simulink model "OperatingMode_PLCCoder"  (R2024b)
settings: Solver=FixedStepAuto  StartTime=0.0  StopTime=2  FixedStep=0.1  MaxStep=TsModel  RelTol=1e-3
undefined symbols (not defined in the file): operatingMode
libraries: simulink x3
settings Model: DataDictionary=LocalDataD_SupervisoryLogic.sldd  Creator=vlenzi  LastModifiedBy=vlenzi
settings SolverCC: AlgebraicLoopSolver=TrustRegion
settings OptimizationCC: DefaultParameterBehavior=Inlined  ReuseModelBlockBuffer=off
settings DebuggingCC: InheritedTsInSrcMsg=none  UnconnectedInputMsg=warning  UnconnectedOutputMsg=warning  UnconnectedLineMsg=warning
settings ModelReferenceCC: EnableRefExpFcnMdlSchedulingChecks=on
settings RTWCC: GPUComputeCapability=3.5  DLArmComputeVersion=19.05
settings ConfigComp: PLC_OutputDir=..\Code\plcsrc  PLC_TargetIDE=twincat3  PLC_GenerateTestbench=on  PLC_GenerateTestbenchDiagCode=on  PLC_MultiTBSigbuilderTimeRange=off  PLC_GenerateReusableCode=on  PLC_InlineNamedConstant=on  PLC_FoldFBCallOutputVar=on  PLC_RemoveUnusedSSMethodCallArguments=on  PLC_FBUseSubsystemInstanceName=on  PLC_RemoveTopFBSSMethodType=on  PLC_UseCallOutputArgSyntax=off  PLC_OverrideDefaultNameLength=on  PLC_EnableUnsignedAndDoubleTypes=off  PLC_EnableUDTSplitting=off  PLC_MaxFieldsInUDT=500  PLC_GenerateEnumCastFunction=on  PLC_InlineEnumCastFunction=off  PLC_RTWMaxIdLength=64  PLC_GenerateWebView=on

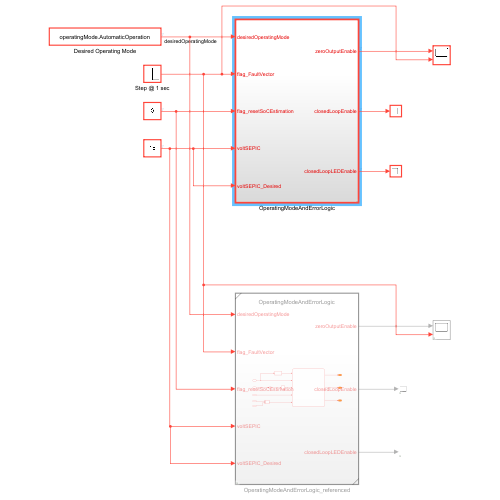
[thumbnail: Simulink's stored preview of the top-level diagram]
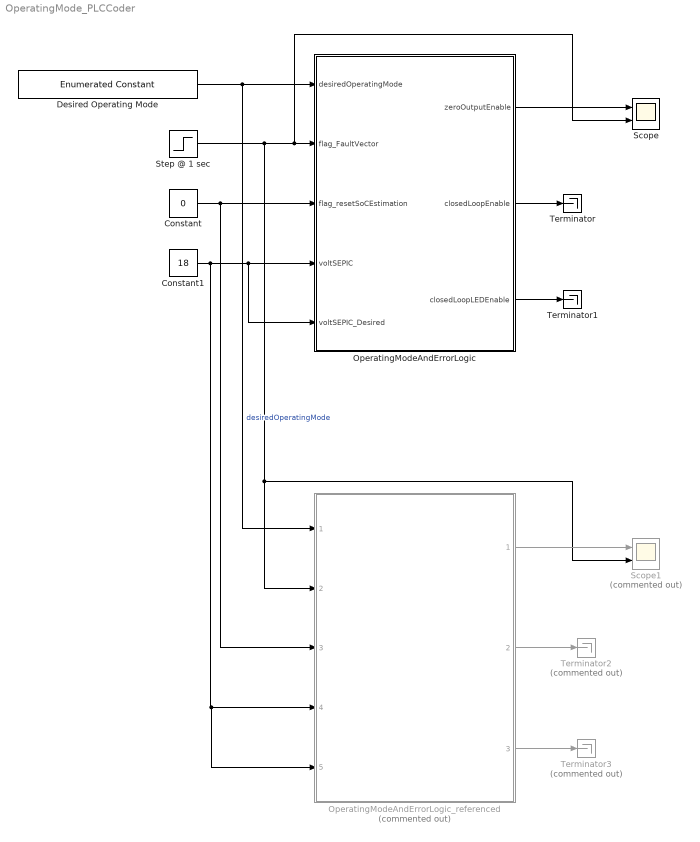
== system OperatingMode_PLCCoder ==
  Constant : Constant  Value=0  OutDataTypeStr=boolean  SampleTime=-1
  Constant1 : Constant  Value=18  SampleTime=-1
  Desired Operating Mode : simulink/Sources/Enumerated Constant  OutDataTypeStr=Enum: operatingMode  Value=operatingMode.AutomaticOperation  SampleTime=-1
  OperatingModeAndErrorLogic : Subsystem  TreatAsAtomicUnit=on
  OperatingModeAndErrorLogic_referenced : Subsystem  Commented=on  TreatAsAtomicUnit=on  ReferencedSubsystem=OperatingModeAndErrorLogic
  Scope : Scope  NumInputPorts=2
  Scope1 : Scope  Commented=on  NumInputPorts=2
  Step @ 1 sec : Step  Before=1  After=0
  Terminator : Terminator
  Terminator1 : Terminator
  Terminator2 : Terminator  Commented=on
  Terminator3 : Terminator  Commented=on
  wires:
  Step @ 1 sec/1 -> Scope1/2, OperatingModeAndErrorLogic_referenced/2, Scope/2, OperatingModeAndErrorLogic/2(flag_FaultVector)
  Desired Operating Mode/1 -> OperatingModeAndErrorLogic_referenced/1, OperatingModeAndErrorLogic/1(desiredOperatingMode)  "desiredOperatingMode"
  Constant/1 -> OperatingModeAndErrorLogic_referenced/3, OperatingModeAndErrorLogic/3(flag_resetSoCEstimation)
  Constant1/1 -> OperatingModeAndErrorLogic_referenced/5, OperatingModeAndErrorLogic_referenced/4, OperatingModeAndErrorLogic/5(voltSEPIC_Desired), OperatingModeAndErrorLogic/4(voltSEPIC)
  OperatingModeAndErrorLogic/1(zeroOutputEnable) -> Scope/1
  OperatingModeAndErrorLogic/2(closedLoopEnable) -> Terminator/1
  OperatingModeAndErrorLogic/3(closedLoopLEDEnable) -> Terminator1/1
  OperatingModeAndErrorLogic_referenced/1 -> Scope1/1
  OperatingModeAndErrorLogic_referenced/2 -> Terminator2/1
  OperatingModeAndErrorLogic_referenced/3 -> Terminator3/1

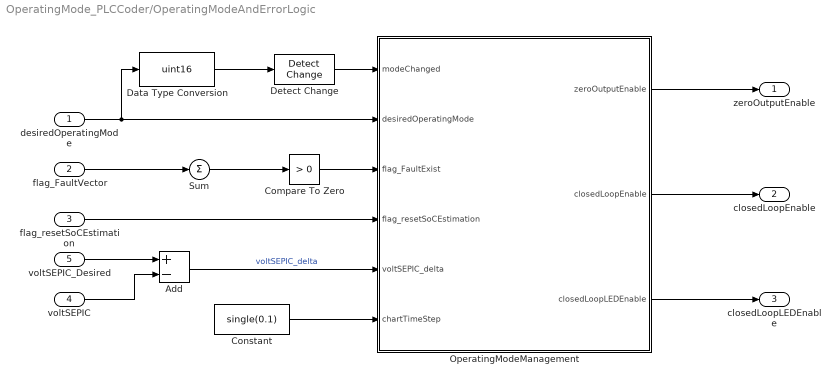
== system OperatingMode_PLCCoder/OperatingModeAndErrorLogic ==
  desiredOperatingMode : Inport
  flag_FaultVector : Inport  Port=2
  flag_resetSoCEstimation : Inport  Port=3
  voltSEPIC : Inport  Port=4
  voltSEPIC_Desired : Inport  Port=5
  Add : Sum  Inputs=+-
  Compare To Zero : simulink/Logic and Bit Operations/Compare To Zero  relop=>  OutDataTypeStr=boolean
  Constant : Constant  Value=single(0.1)  OutDataTypeStr=single  SampleTime=-1
  Data Type Conversion : DataTypeConversion  OutDataTypeStr=uint16  SaturateOnIntegerOverflow=off  RndMeth=Floor
  Detect Change : simulink/Logic and Bit Operations/Detect Change  vinit=0  OutDataTypeStr=boolean
  OperatingModeManagement : Stateflow chart  TreatAsAtomicUnit=on
  Sum : Sum  Inputs=+
  zeroOutputEnable : Outport  OutDataTypeStr=boolean  Unit=1  PortDimensions=1
  closedLoopEnable : Outport  Port=2  OutDataTypeStr=boolean  Unit=1  PortDimensions=1
  closedLoopLEDEnable : Outport  Port=3  OutDataTypeStr=boolean  Unit=1  PortDimensions=1
  wires:
  Compare To Zero/1 -> OperatingModeManagement/3(flag_FaultExist)
  Sum/1 -> Compare To Zero/1
  OperatingModeManagement/3(closedLoopLEDEnable) -> closedLoopLEDEnable/1
  OperatingModeManagement/2(closedLoopEnable) -> closedLoopEnable/1
  flag_resetSoCEstimation/1 -> OperatingModeManagement/4(flag_resetSoCEstimation)
  OperatingModeManagement/1(zeroOutputEnable) -> zeroOutputEnable/1
  Data Type Conversion/1 -> Detect Change/1
  Detect Change/1 -> OperatingModeManagement/1(modeChanged)
  flag_FaultVector/1 -> Sum/1
  desiredOperatingMode/1 -> Data Type Conversion/1, OperatingModeManagement/2(desiredOperatingMode)
  voltSEPIC_Desired/1 -> Add/1
  voltSEPIC/1 -> Add/2
  Add/1 -> OperatingModeManagement/5(voltSEPIC_delta)  "voltSEPIC_delta"
  Constant/1 -> OperatingModeManagement/6(chartTimeStep)

== stateflow chart OperatingMode_PLCCoder/OperatingModeAndErrorLogic/OperatingModeManagement ==
  state Operation
    state CheckingFault [parallel]
      settings: executionOrder=1
      state SystemKO
        en:zeroOutputEnable=true;
      state SystemOK
        en:zeroOutputEnable=false;
      (default) -> SystemKO
      SystemOK -> SystemKO : [flag_FaultExist]
      SystemKO -> SystemOK : [~flag_FaultExist]
    state OperatingMode [parallel]
      settings: executionOrder=2
      state AllOpenLoop
        en:closedLoopEnable=false;
        en:closedLoopLEDEnable=false;
      state VoltOpen_CurrClosed
        en:closedLoopEnable=false;
        en:closedLoopLEDEnable=true;
      state VoltClosed_CurrOpen
        en:closedLoopEnable=true;
        en:closedLoopLEDEnable=false;
      state AllClosedLoop
        en:closedLoopEnable=true;
        en:closedLoopLEDEnable=true;
      state AutomaticOperation
        state AllOpenLoop
          en:closedLoopEnable=false;
          en:closedLoopLEDEnable=false;
          en:counter=0;
        state WaitingForVoltageSettling
          en:closedLoopEnable=false;
          en:closedLoopLEDEnable=false;
          du:counter=counter+1;
        state AllClosedLoop
          en:closedLoopEnable=true;
          en:closedLoopLEDEnable=true;
        (default) -> Operation.OperatingMode.AutomaticOperation.AllOpenLoop
        Operation.OperatingMode.AutomaticOperation.AllOpenLoop -> WaitingForVoltageSettling : [abs(voltSEPIC_delta) <=1]
        WaitingForVoltageSettling -> Operation.OperatingMode.AutomaticOperation.AllOpenLoop [order 2] : [abs(voltSEPIC_delta) >1.5]
        WaitingForVoltageSettling -> Operation.OperatingMode.AutomaticOperation.AllClosedLoop [order 1] : [counter>floor(2/chartTimeStep)]
      state NoOutput
        en:zeroOutputEnable=true;
      (default) -> (junction 91)
      (junction 91) -> Operation.OperatingMode.AllOpenLoop [order 1] : [desiredOperatingMode==AllOpenLoop]
      Operation.OperatingMode.AllOpenLoop -> OperatingMode : [modeChanged]
      (junction 91) -> (junction 92) [order 2]
      (junction 92) -> VoltOpen_CurrClosed [order 1] : [desiredOperatingMode==VoltOpen_CurrClosed]
      VoltOpen_CurrClosed -> OperatingMode : [modeChanged]
      (junction 92) -> (junction 93) [order 2]
      VoltClosed_CurrOpen -> OperatingMode : [modeChanged]
      (junction 93) -> VoltClosed_CurrOpen [order 1] : [desiredOperatingMode==VoltClosed_CurrOpen]
      (junction 93) -> (junction 94) [order 2]
      (junction 94) -> Operation.OperatingMode.AllClosedLoop [order 1] : [desiredOperatingMode==AllClosedLoop]
      Operation.OperatingMode.AllClosedLoop -> OperatingMode : [modeChanged]
      (junction 94) -> (junction 127) [order 2]
      (junction 127) -> AutomaticOperation [order 1] : [desiredOperatingMode==AutomaticOperation]
      (junction 127) -> NoOutput [order 2]
      AutomaticOperation -> OperatingMode : [modeChanged]
      NoOutput -> OperatingMode : [modeChanged]
  state Initialization_no_output
    en:closedLoopEnable=false;
    en:closedLoopLEDEnable=false;
    en:zeroOutputEnable=true;
  (default) -> Initialization_no_output
  Initialization_no_output -> Operation : [desiredOperatingMode ~= NoOutput &&flag_resetSoCEstimation==0 ]
  data: modeChanged input boolean; zeroOutputEnable output boolean size=1; desiredOperatingMode input Enum: operatingMode; closedLoopEnable output boolean size=1; closedLoopLEDEnable output boolean size=1; flag_FaultExist input boolean; flag_resetSoCEstimation input boolean; voltSEPIC_delta input; chartTimeStep input; counter local
